simulink model "lotka2_sim"  (Simulink 7.6)
settings: Solver=ode5  StartTime=0.0  StopTime=40  FixedStep=0.01  RelTol=1e-3
values from neighbouring files (symbols this model uses):
  e = 0.2    [lotka2punti_eq.m]
  e1 = 40    [lotka2punti_eq.m]
  e2 = 20    [lotka2punti_eq.m]
  k1 = 150    [lotka2punti_eq.m]
  p = 0.3    [lotka2punti_eq.m]
  x0 = [25,10]'    [lotka2punti_eq.m]
settings Model: Creator=enrico  LastModifiedBy=patrizio
settings OptimizationCC: BooleanDataType=off  InlineInvariantSignals=on  InitFltsAndDblsToZero=on
settings DebuggingCC: SaveWithParameterizedLinksMsg=none  SignalResolutionControl=TryResolveAllWithWarning  SolverPrmCheckMsg=none  MultiTaskDSMMsg=warning  MultiTaskCondExecSysMsg=none  StrictBusMsg=None
settings HardwareCC: TargetUnknown=on
settings RTWCC: IncludeERTFirstTime=on
settings GRTTargetCC: TargetFcnLib=ansi_tfl_tmw.mat

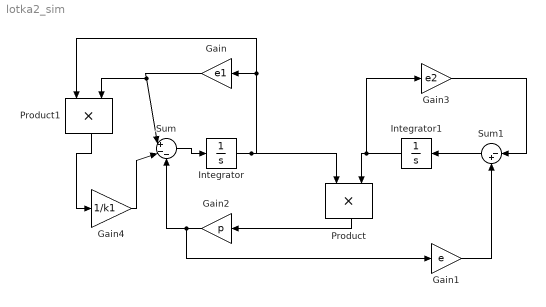
== system lotka2_sim ==
  Gain : Gain  Gain=e1  SaturateOnIntegerOverflow=on  OutDataTypeStr=Inherit: Same as input  ParamDataTypeStr=Inherit: Same as input
  Gain1 : Gain  Gain=e  SaturateOnIntegerOverflow=on  OutDataTypeStr=Inherit: Same as input  ParamDataTypeStr=Inherit: Same as input
  Gain2 : Gain  Gain=p  SaturateOnIntegerOverflow=on  OutDataTypeStr=Inherit: Same as input  ParamDataTypeStr=Inherit: Same as input
  Gain3 : Gain  Gain=e2  SaturateOnIntegerOverflow=on  OutDataTypeStr=Inherit: Same as input  ParamDataTypeStr=Inherit: Same as input
  Gain4 : Gain  Gain=1/k1  SaturateOnIntegerOverflow=on  OutDataTypeStr=Inherit: Same as input  ParamDataTypeStr=Inherit: Same as input
  Integrator : Integrator  InitialCondition=x0(1)
  Integrator1 : Integrator  InitialCondition=x0(2)
  Product : Product  SaturateOnIntegerOverflow=on  RndMeth=Zero  InputSameDT=on  OutDataTypeStr=Inherit: Same as first input
  Product1 : Product  SaturateOnIntegerOverflow=on  RndMeth=Zero  InputSameDT=on  OutDataTypeStr=Inherit: Same as first input
  Sum : Sum  Inputs=|+--  SaturateOnIntegerOverflow=on  InputSameDT=on  OutDataTypeStr=Inherit: Same as first input
  Sum1 : Sum  Inputs=|-+  SaturateOnIntegerOverflow=on  InputSameDT=on  OutDataTypeStr=Inherit: Same as first input
  wires:
  Sum/1 -> Integrator/1
  Sum1/1 -> Integrator1/1
  Integrator/1 -> Product/1, Gain/1, Product1/1
  Gain/1 -> Sum/1, Product1/2
  Integrator1/1 -> Product/2, Gain3/1
  Product/1 -> Gain2/1
  Gain2/1 -> Gain1/1, Sum/3
  Gain1/1 -> Sum1/2
  Gain3/1 -> Sum1/1
  Product1/1 -> Gain4/1
  Gain4/1 -> Sum/2
